simulink library "CompartmentsLib"  (Simulink 7.7)
settings: Solver=ode45  SolverMode=SingleTasking  StartTime=0.0  StopTime=10.0  RelTol=1e-3
undefined symbols (not defined in the file or in its folder): C, d, EK, EL, ENa, gA, gK, gL, gNa, L, magnitude, PSoma1, V0, VR
libraries: CurrentsLib x11, simulink x5, CompartmentsLib x2
settings Model: Creator=jpalma  LastModifiedBy=jpalma

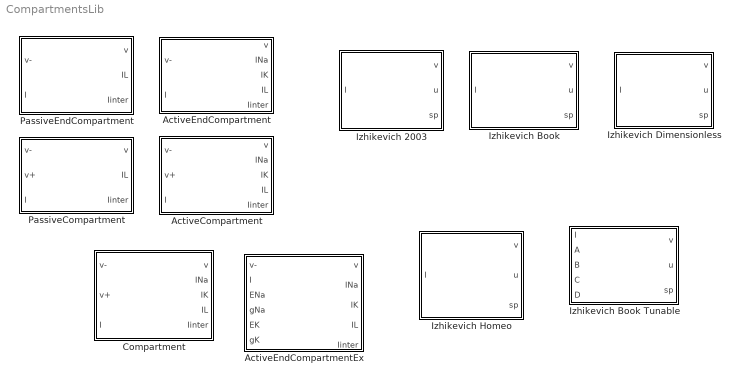
== system CompartmentsLib ==
  ActiveCompartment : Subsystem  mask{C=PSoma1(1), V0=PSoma1(2), gA=PSoma1(9), d=PSoma1(10), L=PSoma1(11), gNa=PSoma1(3), ENa=PSoma1(4), gK=PSoma1(5), EK=PSoma1(6), gL=PSoma1(7), EL=PSoma1(8)}
      mask prompts: C "Capacitance, C"; V0 "Initial Voltage, V0"; gA "Axial Conductance, gA"; d "Comp Diameter, d"; L "Comp Length, L"; gNa "Na Conductance, gNa"; ENa "Na Eq Voltage, ENa"; gK "K Conductance, gK"; EK "K Eq Voltage, EK"; gL "Leak Conductance, gL"; EL "Leak Eq Voltage, EL"
      mask help: Author: Jesse Palma
      mask Help: Author: Jesse Palma
      mask TabNameString: Basics,Basics,Basics,Basics,Basics,Currents,Currents,Currents,Currents,Currents,Currents
      mask Display: image(imread('../Libs/icons/Compartment.jpg'),'center');
  ActiveEndCompartment : Subsystem  mask{C=C, V0=V0, gA=gA, d=d, L=L, gNa=gNa, ENa=ENa, gK=gK, EK=EK, gL=gL, EL=EL}
      mask prompts: C "Capacitance, C"; V0 "Initial Voltage, V0"; gA "Axial Conductance, gA"; d "Comp Diameter, d"; L "Comp Length, L"; gNa "Na Conductance, gNa"; ENa "Na Eq Voltage, ENa"; gK "K Conductance, gK"; EK "K Eq Voltage, EK"; gL "Leak Conductance, gL"; EL "Leak Eq Voltage, EL"
      mask help: Author: Jesse Palma
      mask Help: Author: Jesse Palma
      mask TabNameString: Basic,Basic,Basic,Basic,Basic,Currents,Currents,Currents,Currents,Currents,Currents
      mask Display: image(imread('../Libs/icons/Compartment.jpg'),'center');
  ActiveEndCompartmentEx : Subsystem  mask{C=C, V0=V0, gA=gA, d=d, L=L, gL=gL, EL=EL}
      mask prompts: C "Capacitance, C"; V0 "Initial Voltage, V0"; gA "Axial Conductance, gA"; d "Comp Diameter, d"; L "Comp Length, L"; gL "Leak Conductance, gL"; EL "Leak Eq Voltage, EL"
      mask help: Author: Jesse Palma
      mask Help: Author: Jesse Palma
      mask TabNameString: Basic,Basic,Basic,Basic,Basic,Currents,Currents
      mask Display: image(imread('../Libs/icons/Compartment.jpg'),'center');
  Compartment : Subsystem  BlockChoice=ActiveEndCompartment  mask{ifEnd=on, ifActive=on, settings=UserDefined, C=1, V0=-65, gNa=45, ENa=50, gK=16, EK=-100, gL=0.03, EL=-60, gA=0.25, d=0.06, L=0.4}
      mask prompts: ifEnd "End Compartment"; ifActive "Active Compartment (Na and K)"; settings "Parameters Settings"; C "Capacitance"; V0 "Initial Voltage"; gNa "Na Conductance"; ENa "Na Eq Voltage"; gK "K Conductance"; EK "K Eq Voltage"; gL "Leak Conductance"; EL "Leak Eq Voltage"; gA "Axial Conductance"; d "Compartment Diameter"; L "Compartment Length"
      mask help: Author: Jesse Palma
      mask init:
      | maskStr = get_param(gcb,'MaskValues');
      | if (ifActive)
      |     if (ifEnd)
      |         BlockChoice = 'ActiveEndCompartment';
      |     else
      |         BlockChoice = 'ActiveCompartment';
      |     end
      | else
      |     if (ifEnd)
      |         BlockChoice = 'PassiveEndCompartment';
      |     else
      |         BlockChoice = 'PassiveCompartment';
      |     end
      | end
      | set_param([gcb], 'BlockChoice', BlockChoice);
      settings: TemplateBlock=self  MemberBlocks=ActiveCompartment,ActiveEndCompartment,PassiveCompartment,PassiveEndCompartment
      mask Help: Author: Jesse Palma
      mask StyleString: checkbox,checkbox,popup(Default1|UserDefined),edit,edit,edit,edit,edit,edit,edit,edit,edit,edit,edit
      mask CallbackString:
      | |maskStr = get_param(gcb,'MaskValues');
      | if strcmp(maskStr{2},'on')
      |     set_param(gcb,'MaskVisibilities',{'on';'on';'on';'on';'on';'on';'on';'on';'on';'on';'on';'on';'on';'on'});
      | else
      |     set_param(gcb,'MaskVisibilities',{'on';'on';'on';'on';'on';'off';'off';'off';'off';'on';'on';'on';'on';'on'});
      | end|maskStr = get_param(gcb,'MaskValues');
      | if strcmp(maskStr{3},'Default1')
      |    maskStr = get_param(gcb,'MaskValues');
      |    maskStr{4} = '1';
      |    maskStr{5} = '-65';
      |    maskStr{6} = '45';
      |    maskStr{7} = '50';
      |    maskStr{8} = '16';
      |    maskStr{9} = '-100';
      |    maskStr{10} = '0.03';
      |    maskStr{11} = '-60';
      |    maskStr{12} = '0.25';
      |    maskStr{13} = '0.06';
      |    maskStr{14} = '0.4';
      |    set_param(gcb, 'MaskValues', maskStr);
      | else
      | end|maskStr = get_param(gcb,'MaskValues');
      | maskStr{3} = 'UserDefined';
      | set_param(gcb, 'MaskValues', maskStr);|maskStr = get_param(gcb,'MaskValues');
      | maskStr{3} = 'UserDefined';
      | set_param(gcb, 'MaskValues', maskStr);|maskStr = get_param(gcb,'MaskValues');
      | maskStr{3} = 'UserDefined';
      | set_param(gcb, 'MaskValues', maskStr);|maskStr = get_param(gcb,'MaskValues');
      | maskStr{3} = 'UserDefined';
      | set_param(gcb, 'MaskValues', maskStr);|maskStr = get_param(gcb,'MaskValues');
      | maskStr{3} = 'UserDefined';
      | set_param(gcb, 'MaskValues', maskStr);|maskStr = get_param(gcb,'MaskValues');
      | maskStr{3} = 'UserDefined';
      | set_param(gcb, 'MaskValues', maskStr);|maskStr = get_param(gcb,'MaskValues');
      | maskStr{3} = 'UserDefined';
      | set_param(gcb, 'MaskValues', maskStr);|maskStr = get_param(gcb,'MaskValues');
      | maskStr{3} = 'UserDefined';
      | set_param(gcb, 'MaskValues', maskStr);|maskStr = get_param(gcb,'MaskValues');
      | maskStr{3} = 'UserDefined';
      | set_param(gcb, 'MaskValues', maskStr);|maskStr = get_param(gcb,'MaskValues');
      | maskStr{3} = 'UserDefined';
      | set_param(gcb, 'MaskValues', maskStr);|maskStr = get_param(gcb,'MaskValues');
      | maskStr{3} = 'UserDefined';
      | set_param(gcb, 'MaskValues', maskStr);
      mask TabNameString: Basics,Basics,Basics,Basics,Basics,Currents,Currents,Currents,Currents,Currents,Currents,Geometry,Geometry,Geometry
      mask Display: image(imread('../Libs/icons/Compartment.jpg'),'center');
  Izhikevich 2003 : Subsystem  mask{settings=UserDefined, A=0.02, B=0.2, C=-65, D=8, P2=0.04, P1=5, P0=140, VP=30, V0=-70, U0=-20}
      mask prompts: settings "Parameter Settings"; A "a, recovery u time constant"; B "b, dynamics parameter"; C "c,  reset value v"; D "d, reset shift u"; P2 "P2, 2nd order term"; P1 "P1, 1st order term"; P0 "P0, constant term"; VP "Vp, voltage peak"; V0 "V0, initial v value"; U0 "U0, intial u value"
      mask help:
      | Model from Eugene Izhikevich's 2003 Paper
      |     (Equations 1, 2 & 3)
      | Also in Eugene Izhikevich's 2004 Paper
      |
      | Simulink Model Design: Jesse Palma
      mask init:
      | maskStr = get_param(gcb,'MaskValues');
      mask Help:
      | Model from Eugene Izhikevich's 2003 Paper
      | <br>(Equations 1, 2 & 3)
      | <br>Also in Eugene Izhikevich's 2004 Paper
      | <br><br>
      | Simulink Model Design: Jesse Palma
      mask StyleString: popup(Tonic-Spiking-I04|Phasic-Spiking-I04|Tonic-Bursting-I04|UserDefined),edit,edit,edit,edit,edit,edit,edit,edit,edit,edit
      mask CallbackString:
      | maskStr = get_param(gcb,'MaskValues');
      | if strcmp(maskStr{1},'Tonic-Spiking-I04')
      |    maskStr = get_param(gcb,'MaskValues');
      |    maskStr{2} = '0.02'; %A
      |    maskStr{3} = '0.2';  %B
      |    maskStr{4} = '-65';  %C
      |    maskStr{5} = '6';    %D
      |    maskStr{6} = '0.04'; %P2
      |    maskStr{7} = '5';    %P1
      |    maskStr{8} = '140';  %P0
      |    maskStr{9} = '30';   %VP
      |    maskStr{10} = '-70'; %V0
      |    maskStr{11} = '-20';  %U0
      |    set_param(gcb, 'MaskValues', maskStr);
      | end
      | if strcmp(maskStr{1},'Phasic-Spiking-I04')
      |    maskStr = get_param(gcb,'MaskValues');
      |    maskStr{2} = '0.02'; %A
      |    maskStr{3} = '0.25';  %B
      |    maskStr{4} = '-65';  %C
      |    maskStr{5} = '6';    %D
      |    maskStr{6} = '0.04'; %P2
      |    maskStr{7} = '5';    %P1
      |    maskStr{8} = '140';  %P0
      |    maskStr{9} = '30';   %VP
      |    maskStr{10} = '-70'; %V0
      |    maskStr{11} = '-20';  %U0
      |    set_param(gcb, 'MaskValues', maskStr);
      | end
      | if strcmp(maskStr{1},'Tonic-Bursting-I04')
      |    maskStr = get_param(gcb,'MaskValues');
      |    maskStr{2} = '0.02'; %A
      |    maskStr{3} = '0.2';  %B
      |    maskStr{4} = '-50';  %C
      |    maskStr{5} = '2';    %D
      |    maskStr{6} = '0.04'; %P2
      |    maskStr{7} = '5';    %P1
      |    maskStr{8} = '140';  %P0
      |    maskStr{9} = '30';   %VP
      |    maskStr{10} = '-70'; %V0
      |    maskStr{11} = '-20';  %U0
      |    set_param(gcb, 'MaskValues', maskStr);
      | end|maskStr = get_param(gcb,'MaskValues');
      | maskStr{1} = 'UserDefined';
      | set_param(gcb, 'MaskValues', maskStr);|maskStr = get_param(gcb,'MaskValues');
      | maskStr{1} = 'UserDefined';
      | set_param(gcb, 'MaskValues', maskStr);|maskStr = get_param(gcb,'MaskValues');
      | maskStr{1} = 'UserDefined';
      | set_param(gcb, 'MaskValues', maskStr);|maskStr = get_param(gcb,'MaskValues');
      | maskStr{1} = 'UserDefined';
      | set_param(gcb, 'MaskValues', maskStr);|maskStr = get_param(gcb,'MaskValues');
      | maskStr{1} = 'UserDefined';
      | set_param(gcb, 'MaskValues', maskStr);|maskStr = get_param(gcb,'MaskValues');
      | maskStr{1} = 'UserDefined';
      | set_param(gcb, 'MaskValues', maskStr);|maskStr = get_param(gcb,'MaskValues');
      | maskStr{1} = 'UserDefined';
      | set_param(gcb, 'MaskValues', maskStr);|maskStr = get_param(gcb,'MaskValues');
      | maskStr{1} = 'UserDefined';
      | set_param(gcb, 'MaskValues', maskStr);|maskStr = get_param(gcb,'MaskValues');
      | maskStr{1} = 'UserDefined';
      | set_param(gcb, 'MaskValues', maskStr);|maskStr = get_param(gcb,'MaskValues');
      | maskStr{1} = 'UserDefined';
      | set_param(gcb, 'MaskValues', maskStr);
      mask Display: image(imread('../Libs/icons/Izhik.jpg'),'center');
  Izhikevich Book : Subsystem  mask{settings=UserDefined, A=0.03, B=-2, C=-50, D=100, CP=100, K=0.7, VR=-60, VT=-40, VP=35, V0=-60, U0=0}
      mask prompts: settings "Parameter Settings"; A "a, recovery u time constant"; B "b, dynamics parameter"; C "c,  reset value v"; D "d, reset shift u"; CP "Cp, capacitance"; VR "Vr, voltage rest"; VT "Vt, voltage threshold"; VP "Vpeak, voltage peak reset"; V0 "V0, initial v value"; U0 "U0, initial u value"
      mask help:
      | Model from Eugene Izhikevich's book "Dynamical Systems in Neuroscience"
      |     (Equations 8.5 & 8.6 on page 273)
      | 9 Paramters are reducable to 4-parameter model.
      |
      | Simulink Model Design: Jesse Palma
      mask Help:
      | Model from Eugene Izhikevich's book
      | <a href=http://www.izhikevich.org/publications/dsn/index.htm>"Dynamical Systems in Neuroscience"</a>
      | <br>(Equations 8.5 & 8.6 on page 273)<br>
      | 9 Paramters are reducable to 4-parameter model.
      | <br><br>
      | Simulink Model Design: Jesse Palma
      mask StyleString: popup(Regular-Spiking(p274-283)|Motor(p287)|UserDefined),edit,edit,edit,edit,edit,edit,edit,edit,edit,edit,edit
      mask CallbackString:
      | maskStr = get_param(gcb,'MaskValues');
      | if strcmp(maskStr{1},'Regular-Spiking(p274-283)')
      |    maskStr = get_param(gcb,'MaskValues');
      |    maskStr{2} = '0.03'; %A
      |    maskStr{3} = '-2';   %B
      |    maskStr{4} = '-50';  %C
      |    maskStr{5} = '100';  %D
      |    maskStr{6} = '100';  %CP
      |    maskStr{7} = '0.7';  %K
      |    maskStr{8} = '-60';  %VR
      |    maskStr{9} = '-40';  %VT
      |    maskStr{10} = '35';  %VP
      |    maskStr{11} = '-60'; %V0
      |    maskStr{12} = '0';   %U0
      |    set_param(gcb, 'MaskValues', maskStr);
      | end
      | if strcmp(maskStr{1},'Motor(p287)')
      |    maskStr = get_param(gcb,'MaskValues');
      |    maskStr{2} = '0.01'; %A
      |    maskStr{3} = '-0.25';%B
      |    maskStr{4} = '-40';  %C
      |    maskStr{5} = '90';   %D
      |    maskStr{6} = '30';   %CP
      |    maskStr{7} = '3';    %K
      |    maskStr{8} = '-55';  %VR
      |    maskStr{9} = '-42';  %VT
      |    maskStr{10} = '10';  %VP
      |    maskStr{11} = '-55'; %V0
      |    maskStr{12} = '0';   %U0
      |    set_param(gcb, 'MaskValues', maskStr);
      | end|maskStr = get_param(gcb,'MaskValues');
      | maskStr{1} = 'UserDefined';
      | set_param(gcb, 'MaskValues', maskStr);|maskStr = get_param(gcb,'MaskValues');
      | maskStr{1} = 'UserDefined';
      | set_param(gcb, 'MaskValues', maskStr);|maskStr = get_param(gcb,'MaskValues');
      | maskStr{1} = 'UserDefined';
      | set_param(gcb, 'MaskValues', maskStr);|maskStr = get_param(gcb,'MaskValues');
      | maskStr{1} = 'UserDefined';
      | set_param(gcb, 'MaskValues', maskStr);|maskStr = get_param(gcb,'MaskValues');
      | maskStr{1} = 'UserDefined';
      | set_param(gcb, 'MaskValues', maskStr);|maskStr = get_param(gcb,'MaskValues');
      | maskStr{1} = 'UserDefined';
      | set_param(gcb, 'MaskValues', maskStr);|maskStr = get_param(gcb,'MaskValues');
      | maskStr{1} = 'UserDefined';
      | set_param(gcb, 'MaskValues', maskStr);|maskStr = get_param(gcb,'MaskValues');
      | maskStr{1} = 'UserDefined';
      | set_param(gcb, 'MaskValues', maskStr);|maskStr = get_param(gcb,'MaskValues');
      | maskStr{1} = 'UserDefined';
      | set_param(gcb, 'MaskValues', maskStr);|maskStr = get_param(gcb,'MaskValues');
      | maskStr{1} = 'UserDefined';
      | set_param(gcb, 'MaskValues', maskStr);|maskStr = get_param(gcb,'MaskValues');
      | maskStr{1} = 'UserDefined';
      | set_param(gcb, 'MaskValues', maskStr);
      mask Display: image(imread('../Libs/icons/Izhik.jpg'),'center');
  "Izhikevich Book Tunable " : Subsystem  mask{settings=UserDefined, A=0.03, B=-2, C=-50, D=100, CP=100, K=0.7, VR=-60, VT=-40, VP=35, V0=-60, U0=0}
      mask prompts: settings "Parameter Settings"; A "a, recovery u time constant"; B "b, dynamics parameter"; C "c,  reset value v"; D "d, reset shift u"; CP "Cp, capacitance"; VR "Vr, voltage rest"; VT "Vt, voltage threshold"; VP "Vpeak, voltage peak reset"; V0 "V0, initial v value"; U0 "U0, initial u value"
      mask help:
      | Model from Eugene Izhikevich's book "Dynamical Systems in Neuroscience"
      |     (Equations 8.5 & 8.6 on page 273)
      | 9 Paramters are reducable to 4-parameter model.
      |
      | Simulink Model Design: Jesse Palma
      mask Help:
      | Model from Eugene Izhikevich's book
      | <a href=http://www.izhikevich.org/publications/dsn/index.htm>"Dynamical Systems in Neuroscience"</a>
      | <br>(Equations 8.5 & 8.6 on page 273)<br>
      | 9 Paramters are reducable to 4-parameter model.
      | <br><br>
      | Simulink Model Design: Jesse Palma
      mask StyleString: popup(Regular-Spiking(p274-283)|Motor(p287)|UserDefined),edit,edit,edit,edit,edit,edit,edit,edit,edit,edit,edit
      mask CallbackString:
      | maskStr = get_param(gcb,'MaskValues');
      | if strcmp(maskStr{1},'Regular-Spiking(p274-283)')
      |    maskStr = get_param(gcb,'MaskValues');
      |    maskStr{2} = '0.03'; %A
      |    maskStr{3} = '-2';   %B
      |    maskStr{4} = '-50';  %C
      |    maskStr{5} = '100';  %D
      |    maskStr{6} = '100';  %CP
      |    maskStr{7} = '0.7';  %K
      |    maskStr{8} = '-60';  %VR
      |    maskStr{9} = '-40';  %VT
      |    maskStr{10} = '35';  %VP
      |    maskStr{11} = '-60'; %V0
      |    maskStr{12} = '0';   %U0
      |    set_param(gcb, 'MaskValues', maskStr);
      | end
      | if strcmp(maskStr{1},'Motor(p287)')
      |    maskStr = get_param(gcb,'MaskValues');
      |    maskStr{2} = '0.01'; %A
      |    maskStr{3} = '-0.25';%B
      |    maskStr{4} = '-40';  %C
      |    maskStr{5} = '90';   %D
      |    maskStr{6} = '30';   %CP
      |    maskStr{7} = '3';    %K
      |    maskStr{8} = '-55';  %VR
      |    maskStr{9} = '-42';  %VT
      |    maskStr{10} = '10';  %VP
      |    maskStr{11} = '-55'; %V0
      |    maskStr{12} = '0';   %U0
      |    set_param(gcb, 'MaskValues', maskStr);
      | end|maskStr = get_param(gcb,'MaskValues');
      | maskStr{1} = 'UserDefined';
      | set_param(gcb, 'MaskValues', maskStr);|maskStr = get_param(gcb,'MaskValues');
      | maskStr{1} = 'UserDefined';
      | set_param(gcb, 'MaskValues', maskStr);|maskStr = get_param(gcb,'MaskValues');
      | maskStr{1} = 'UserDefined';
      | set_param(gcb, 'MaskValues', maskStr);|maskStr = get_param(gcb,'MaskValues');
      | maskStr{1} = 'UserDefined';
      | set_param(gcb, 'MaskValues', maskStr);|maskStr = get_param(gcb,'MaskValues');
      | maskStr{1} = 'UserDefined';
      | set_param(gcb, 'MaskValues', maskStr);|maskStr = get_param(gcb,'MaskValues');
      | maskStr{1} = 'UserDefined';
      | set_param(gcb, 'MaskValues', maskStr);|maskStr = get_param(gcb,'MaskValues');
      | maskStr{1} = 'UserDefined';
      | set_param(gcb, 'MaskValues', maskStr);|maskStr = get_param(gcb,'MaskValues');
      | maskStr{1} = 'UserDefined';
      | set_param(gcb, 'MaskValues', maskStr);|maskStr = get_param(gcb,'MaskValues');
      | maskStr{1} = 'UserDefined';
      | set_param(gcb, 'MaskValues', maskStr);|maskStr = get_param(gcb,'MaskValues');
      | maskStr{1} = 'UserDefined';
      | set_param(gcb, 'MaskValues', maskStr);|maskStr = get_param(gcb,'MaskValues');
      | maskStr{1} = 'UserDefined';
      | set_param(gcb, 'MaskValues', maskStr);
      mask Display: image(imread('../Libs/icons/Izhik.jpg'),'center');
  Izhikevich Dimensionless : Subsystem  mask{settings=UserDefined, A=1, B=1, C=1, D=1, V0=0, U0=0}
      mask prompts: settings "Parameter Settings"; A "a, recovery u time constant"; B "b, dynamics parameter"; C "c,  reset value v"; D "d, reset shift u"; V0 "V0, initial v value"; U0 "U0, initial u value"
      mask help:
      | Dimensionless Model from Eugene Izhikevich's book "Dynamical Systems in Neuroscience"
      |     (Equations 8.3 & 8.4 on page 273)
      |
      | Simulink Model Design: Jesse Palma
      mask init:
      | maskStr = get_param(gcb,'MaskValues');
      mask Help:
      | Dimensionless Model from Eugene Izhikevich's book "Dynamical Systems in Neuroscience"
      |     (Equations 8.3 & 8.4 on page 273)
      | 
      | Simulink Model Design: Jesse Palma
      mask StyleString: popup(Default1|UserDefined),edit,edit,edit,edit,edit,edit
      mask CallbackString:
      | maskStr = get_param(gcb,'MaskValues');
      | if strcmp(maskStr{1},'Default1')
      |    maskStr = get_param(gcb,'MaskValues');
      |    maskStr{2} = '1';
      |    maskStr{3} = '1';
      |    maskStr{4} = '1';
      |    maskStr{5} = '1';
      |    maskStr{6} = '0';
      |    maskStr{7} = '0';
      |    set_param(gcb, 'MaskValues', maskStr);
      | else
      | end|maskStr = get_param(gcb,'MaskValues');
      | maskStr{1} = 'UserDefined';
      | set_param(gcb, 'MaskValues', maskStr);|maskStr = get_param(gcb,'MaskValues');
      | maskStr{1} = 'UserDefined';
      | set_param(gcb, 'MaskValues', maskStr);|maskStr = get_param(gcb,'MaskValues');
      | maskStr{1} = 'UserDefined';
      | set_param(gcb, 'MaskValues', maskStr);|maskStr = get_param(gcb,'MaskValues');
      | maskStr{1} = 'UserDefined';
      | set_param(gcb, 'MaskValues', maskStr);|maskStr = get_param(gcb,'MaskValues');
      | maskStr{1} = 'UserDefined';
      | set_param(gcb, 'MaskValues', maskStr);|maskStr = get_param(gcb,'MaskValues');
      | maskStr{1} = 'UserDefined';
      | set_param(gcb, 'MaskValues', maskStr);
      mask Display: image(imread('../Libs/icons/Izhik.jpg'),'center');
  Izhikevich Homeo : Subsystem
      mask Display: image(imread('../Libs/icons/Izhik.jpg'),'center');
  PassiveCompartment : Subsystem  mask{C=C, V0=V0, gA=gA, d=d, L=L, gL=gL, EL=EL}
      mask prompts: C "Capacitance, C"; V0 "Initial Voltage, V0"; gA "Axial Conductance, gA"; d "Comp Diameter, d"; L "Comp Length, L"; gL "Leak Conductance, gL"; EL "Leak Eq Voltage, EL"
      mask help: Author: Jesse Palma
      mask Help: Author: Jesse Palma
      mask TabNameString: Basics,Basics,Basics,Basics,Basics,Currents,Currents
      mask Display: image(imread('../Libs/icons/Compartment.jpg'),'center');
  PassiveEndCompartment : Subsystem  mask{C=C, V0=V0, gA=gA, d=d, L=L, gL=gL, EL=EL}
      mask prompts: C "Capacitance, C"; V0 "Initial Voltage, V0"; gA "Axial Conductance, gA"; d "Comp Diameter, d"; L "Comp Length, L"; gL "Leak Conductance, gL"; EL "Leak Eq Voltage, EL"
      mask help: Author: Jesse Palma
      mask Help: Author: Jesse Palma
      mask TabNameString: Basic,Basic,Basic,Basic,Basic,Currents,Currents
      mask Display: image(imread('../Libs/icons/Compartment.jpg'),'center');

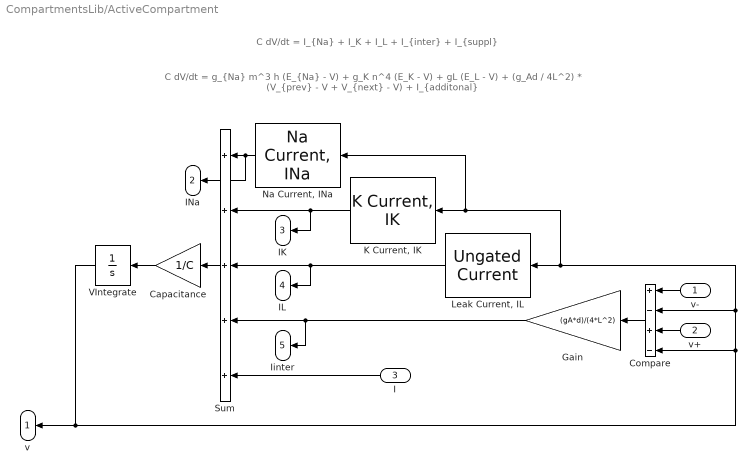
== system CompartmentsLib/ActiveCompartment ==
  note: C dV/dt = I_{Na} + I_K + I_L + I_{inter} + I_{suppl}
  note: C dV/dt = g_{Na} m^3 h (E_{Na} - V) + g_K n^4 (E_K - V) + gL (E_L - V) + (g_Ad / 4L^2) * (V_{prev} - V + V_{next} - V) + I_{additonal}
  v- : Inport
  v+ : Inport  Port=2
  I : Inport  Port=3
  Capacitance : Gain  Gain=1/C
  Compare : Sum  Inputs=+-+-
  Gain : Gain  Gain=(gA*d)/(4*L^2)
  "K Current, IK" : CurrentsLib/K Current, IK  SystemSampleTime=-1  EK=EK  gK=gK  n_a=n3_alpha  n_b=n3_beta
  "Leak Current, IL" : CurrentsLib/Ungated Current  SystemSampleTime=-1  EX=EL  gX=gL
  "Na Current, INa" : CurrentsLib/Na Current, INa  SystemSampleTime=-1  ENa=ENa  gNa=gNa  m_a=m3_alpha  m_b=m3_beta  h_a=h3_alpha  h_b=h3_beta
  Sum : Sum  Inputs=+++++
  VIntegrate : Integrator  InitialCondition=V0
  v : Outport
  INa : Outport  Port=2
  IK : Outport  Port=3
  IL : Outport  Port=4
  Iinter : Outport  Port=5
  wires:
  "K Current, IK"/1 -> IK/1, Sum/2
  "Na Current, INa"/1 -> INa/1, Sum/1
  Gain/1 -> Sum/4, Iinter/1
  I/1 -> Sum/5
  VIntegrate/1 -> v/1, "Na Current, INa"/1, "K Current, IK"/1, "Leak Current, IL"/1, Compare/2, Compare/4
  Capacitance/1 -> VIntegrate/1
  Sum/1 -> Capacitance/1
  "Leak Current, IL"/1 -> IL/1, Sum/3
  Compare/1 -> Gain/1
  v-/1 -> Compare/1
  v+/1 -> Compare/3

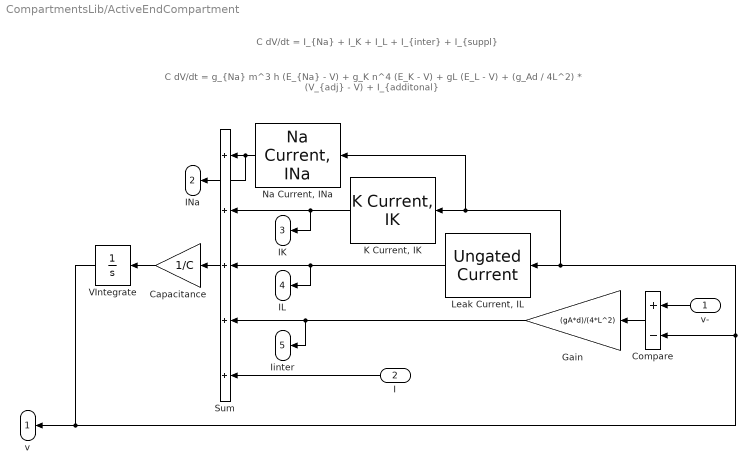
== system CompartmentsLib/ActiveEndCompartment ==
  note: C dV/dt = g_{Na} m^3 h (E_{Na} - V) + g_K n^4 (E_K - V) + gL (E_L - V) + (g_Ad / 4L^2) * (V_{adj} - V) + I_{additonal}
  note: C dV/dt = I_{Na} + I_K + I_L + I_{inter} + I_{suppl}
  v- : Inport
  I : Inport  Port=2
  Capacitance : Gain  Gain=1/C
  Compare : Sum  Inputs=+-
  Gain : Gain  Gain=(gA*d)/(4*L^2)
  "K Current, IK" : CurrentsLib/K Current, IK  SystemSampleTime=-1  EK=EK  gK=gK  n_a=n3_alpha  n_b=n3_beta
  "Leak Current, IL" : CurrentsLib/Ungated Current  SystemSampleTime=-1  EX=EL  gX=gL
  "Na Current, INa" : CurrentsLib/Na Current, INa  SystemSampleTime=-1  ENa=ENa  gNa=gNa  m_a=m3_alpha  m_b=m3_beta  h_a=h3_alpha  h_b=h3_beta
  Sum : Sum  Inputs=+++++
  VIntegrate : Integrator  InitialCondition=V0
  v : Outport
  INa : Outport  Port=2
  IK : Outport  Port=3
  IL : Outport  Port=4
  Iinter : Outport  Port=5
  wires:
  v-/1 -> Compare/1
  Compare/1 -> Gain/1
  "Leak Current, IL"/1 -> Sum/3, IL/1
  Sum/1 -> Capacitance/1
  Capacitance/1 -> VIntegrate/1
  VIntegrate/1 -> v/1, Compare/2, "Leak Current, IL"/1, "K Current, IK"/1, "Na Current, INa"/1
  I/1 -> Sum/5
  Gain/1 -> Iinter/1, Sum/4
  "Na Current, INa"/1 -> Sum/1, INa/1
  "K Current, IK"/1 -> Sum/2, IK/1

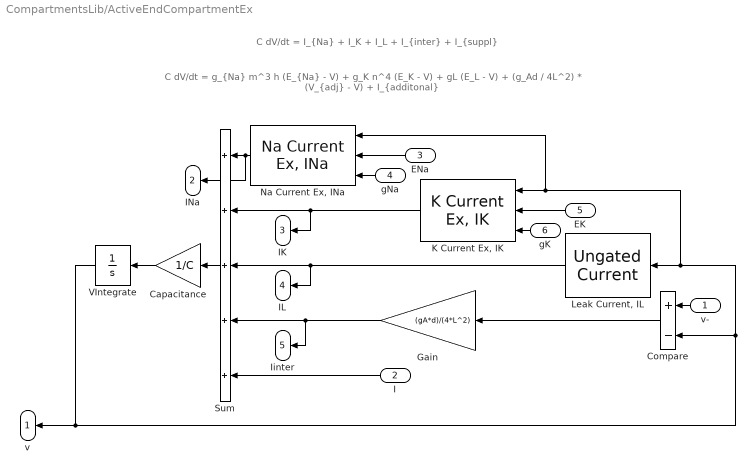
== system CompartmentsLib/ActiveEndCompartmentEx ==
  note: C dV/dt = I_{Na} + I_K + I_L + I_{inter} + I_{suppl}
  note: C dV/dt = g_{Na} m^3 h (E_{Na} - V) + g_K n^4 (E_K - V) + gL (E_L - V) + (g_Ad / 4L^2) * (V_{adj} - V) + I_{additonal}
  v- : Inport
  I : Inport  Port=2
  ENa : Inport  Port=3
  gNa : Inport  Port=4
  EK : Inport  Port=5
  gK : Inport  Port=6
  Capacitance : Gain  Gain=1/C
  Compare : Sum  Inputs=+-
  Gain : Gain  Gain=(gA*d)/(4*L^2)
  "K Current Ex, IK" : CurrentsLib/K Current Ex, IK  SystemSampleTime=-1  n_a=n3_alpha  n_b=n3_beta
  "Leak Current, IL" : CurrentsLib/Ungated Current  SystemSampleTime=-1  EX=EL  gX=gL
  "Na Current Ex, INa" : CurrentsLib/Na Current Ex, INa  SystemSampleTime=-1  m_a=m3_alpha  m_b=m3_beta  h_a=h3_alpha  h_b=h3_beta
  Sum : Sum  Inputs=+++++
  VIntegrate : Integrator  InitialCondition=V0
  v : Outport
  INa : Outport  Port=2
  IK : Outport  Port=3
  IL : Outport  Port=4
  Iinter : Outport  Port=5
  wires:
  "K Current Ex, IK"/1 -> IK/1, Sum/2
  "Na Current Ex, INa"/1 -> INa/1, Sum/1
  Gain/1 -> Sum/4, Iinter/1
  I/1 -> Sum/5
  VIntegrate/1 -> Compare/2, "Leak Current, IL"/1, "K Current Ex, IK"/1, "Na Current Ex, INa"/1, v/1
  Capacitance/1 -> VIntegrate/1
  Sum/1 -> Capacitance/1
  "Leak Current, IL"/1 -> IL/1, Sum/3
  Compare/1 -> Gain/1
  v-/1 -> Compare/1
  ENa/1 -> "Na Current Ex, INa"/2
  gNa/1 -> "Na Current Ex, INa"/3
  gK/1 -> "K Current Ex, IK"/3
  EK/1 -> "K Current Ex, IK"/2

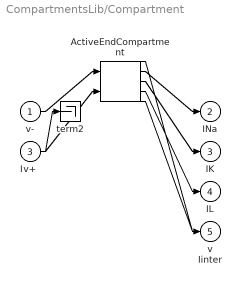
== system CompartmentsLib/Compartment ==
  v- : Inport
  v+ : Inport  Port=2
  I : Inport  Port=3
  ActiveEndCompartment : CompartmentsLib/ActiveEndCompartment  SystemSampleTime=-1  C=PSoma1(1)  V0=PSoma1(2)  gA=PSoma1(9)  d=PSoma1(10)  L=PSoma1(11)  gNa=PSoma1(3)  ENa=PSoma1(4)  gK=PSoma1(5)  EK=PSoma1(6)  gL=PSoma1(7)  EL=PSoma1(8)
  term2 : Terminator
  v : Outport
  INa : Outport  Port=2
  IK : Outport  Port=3
  IL : Outport  Port=4
  Iinter : Outport  Port=5
  wires:
  v-/1 -> ActiveEndCompartment/1
  I/1 -> ActiveEndCompartment/2
  ActiveEndCompartment/1 -> v/1
  ActiveEndCompartment/2 -> INa/1
  ActiveEndCompartment/3 -> IK/1
  ActiveEndCompartment/4 -> IL/1
  ActiveEndCompartment/5 -> Iinter/1
  v+/1 -> term2/1

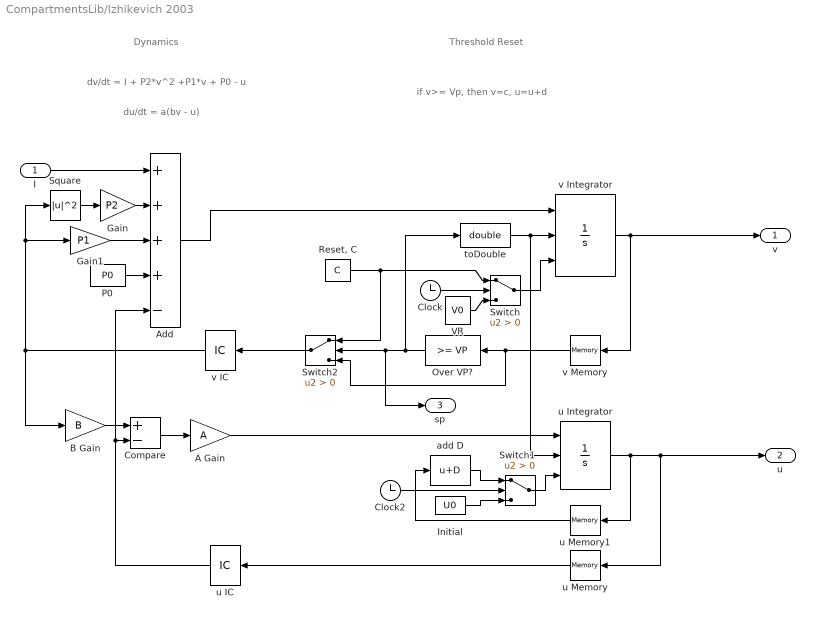
== system CompartmentsLib/Izhikevich 2003 ==
  note: dv/dt = I + P2*v^2 +P1*v + P0 - u
  note: du/dt = a(bv - u)
  note: if v>= Vp, then
      | v=c, u=u+d
  note: Dynamics
  note: Threshold Reset
  I : Inport
  " Initial" : Constant  Value=U0
  A Gain : Gain  Gain=A
  Add : Sum  Inputs=++++-
  B Gain : Gain  Gain=B
  Clock : Clock
      settings: Decimation=10
  Clock2 : Clock
      settings: Decimation=10
  Compare : Sum  Inputs=+-
  Gain : Gain  Gain=P2
  Gain1 : Gain  Gain=P1
  Over VP? : simulink/Logic and Bit Operations/Compare To Constant  SystemSampleTime=-1  relop=>=  const=VP  LogicOutDataTypeMode=boolean  ZeroCross=off
  P0 : Constant  Value=P0
  "Reset, C" : Constant  Value=C
  Square : Math  Operator=magnitude^2  SaturateOnIntegerOverflow=on
  Switch : Switch  Criteria=u2 > Threshold
  Switch1 : Switch  Criteria=u2 > Threshold
  Switch2 : Switch  Criteria=u2 > Threshold
  VR : Constant  Value=V0
  add D : Bias  Bias=D  SaturateOnIntegerOverflow=on
  toDouble : DataTypeConversion  OutDataTypeStr=double
  u IC : InitialCondition  Value=U0
  u Integrator : Integrator  ExternalReset=falling  InitialConditionSource=external
  u Memory : Memory
  u Memory1 : Memory
  v IC : InitialCondition  Value=V0
  v Integrator : Integrator  ExternalReset=rising  InitialConditionSource=external  InitialCondition=VR
  v Memory : Memory
  v : Outport
  u : Outport  Port=2
  sp : Outport  Port=3
  wires:
  u Memory1/1 -> add D/1
  add D/1 -> Switch1/1
  P0/1 -> Add/4
  VR/1 -> Switch/3
  Gain1/1 -> Add/3
  Gain/1 -> Add/2
  Square/1 -> Gain/1
  I/1 -> Add/1
  Add/1 -> v Integrator/1
  A Gain/1 -> u Integrator/1
  B Gain/1 -> Compare/1
  Compare/1 -> A Gain/1
  Over VP?/1 -> toDouble/1, Switch2/2, sp/1
  v Memory/1 -> Over VP?/1, Switch2/3
  " Initial"/1 -> Switch1/3
  Switch1/1 -> u Integrator/3
  Clock2/1 -> Switch1/2
  u Integrator/1 -> u Memory1/1, u Memory/1, u/1
  "Reset, C"/1 -> Switch2/1, Switch/1
  Clock/1 -> Switch/2
  Switch/1 -> v Integrator/3
  v Integrator/1 -> v/1, v Memory/1
  toDouble/1 -> u Integrator/2, v Integrator/2
  Switch2/1 -> v IC/1
  u Memory/1 -> u IC/1
  v IC/1 -> Gain1/1, Square/1, B Gain/1
  u IC/1 -> Add/5, Compare/2

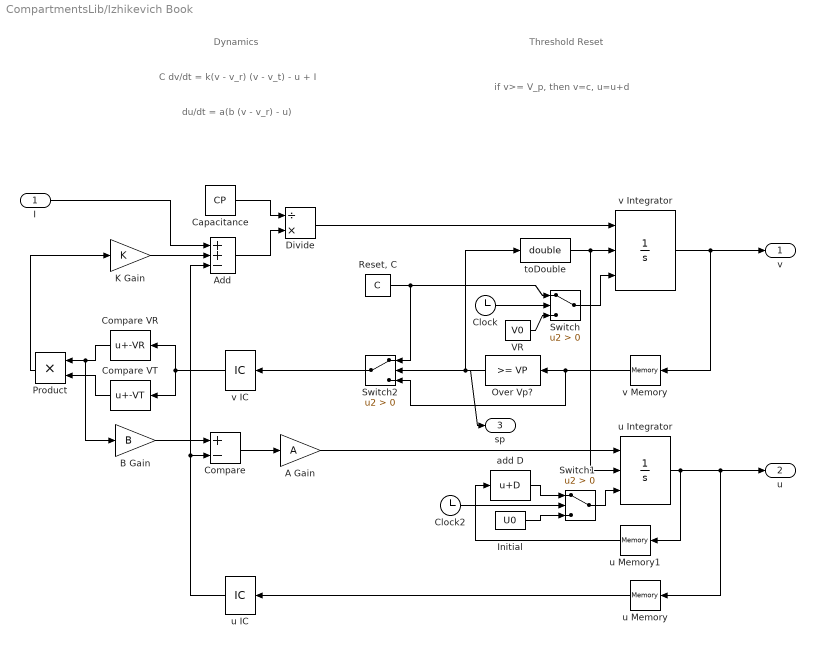
== system CompartmentsLib/Izhikevich Book ==
  note: Threshold Reset
  note: Dynamics
  note: if v>= V_p, then
      | v=c, u=u+d
  note: du/dt = a(b (v - v_r) - u)
  note: C dv/dt = k(v - v_r) (v - v_t) - u + I
  I : Inport
  " Initial" : Constant  Value=U0
  A Gain : Gain  Gain=A
  Add : Sum  Inputs=++-
  B Gain : Gain  Gain=B
  Capacitance : Constant  Value=CP
  Clock : Clock
      settings: Decimation=10
  Clock2 : Clock
      settings: Decimation=10
  Compare : Sum  Inputs=+-
  Compare VR : Bias  Bias=-VR
  Compare VT : Bias  Bias=-VT
  Divide : Product  Inputs=/*
  K Gain : Gain  Gain=K
  Over Vp? : simulink/Logic and Bit Operations/Compare To Constant  SystemSampleTime=-1  relop=>=  const=VP  LogicOutDataTypeMode=boolean  ZeroCross=off
  Product : Product  RndMeth=Zero
  "Reset, C" : Constant  Value=C
  Switch : Switch  Criteria=u2 > Threshold  ZeroCross=off
  Switch1 : Switch  Criteria=u2 > Threshold  ZeroCross=off
  Switch2 : Switch  Criteria=u2 > Threshold  ZeroCross=off
  VR : Constant  Value=V0
  add D : Bias  Bias=D
  toDouble : DataTypeConversion  OutDataTypeStr=double
  u IC : InitialCondition  Value=U0
  u Integrator : Integrator  ExternalReset=rising  InitialConditionSource=external  ZeroCross=off
  u Memory : Memory
  u Memory1 : Memory
  v IC : InitialCondition  Value=V0
  v Integrator : Integrator  ExternalReset=rising  InitialConditionSource=external  InitialCondition=VR  ZeroCross=off
  v Memory : Memory
  v : Outport
  u : Outport  Port=2
  sp : Outport  Port=3
  wires:
  Over Vp?/1 -> toDouble/1, Switch2/2, sp/1
  v Memory/1 -> Over Vp?/1, Switch2/3
  Switch2/1 -> v IC/1
  " Initial"/1 -> Switch1/3
  add D/1 -> Switch1/1
  Switch1/1 -> u Integrator/3
  Clock2/1 -> Switch1/2
  A Gain/1 -> u Integrator/1
  Divide/1 -> v Integrator/1
  u Integrator/1 -> u Memory/1, u/1, u Memory1/1
  "Reset, C"/1 -> Switch/1, Switch2/1
  Clock/1 -> Switch/2
  Switch/1 -> v Integrator/3
  u IC/1 -> Compare/2, Add/3
  v IC/1 -> Compare VR/1, Compare VT/1
  Compare/1 -> A Gain/1
  B Gain/1 -> Compare/1
  u Memory/1 -> u IC/1
  Product/1 -> K Gain/1
  I/1 -> Add/1
  Compare VR/1 -> Product/1, B Gain/1
  Compare VT/1 -> Product/2
  K Gain/1 -> Add/2
  v Integrator/1 -> v Memory/1, v/1
  toDouble/1 -> u Integrator/2, v Integrator/2
  Add/1 -> Divide/2
  Capacitance/1 -> Divide/1
  VR/1 -> Switch/3
  u Memory1/1 -> add D/1

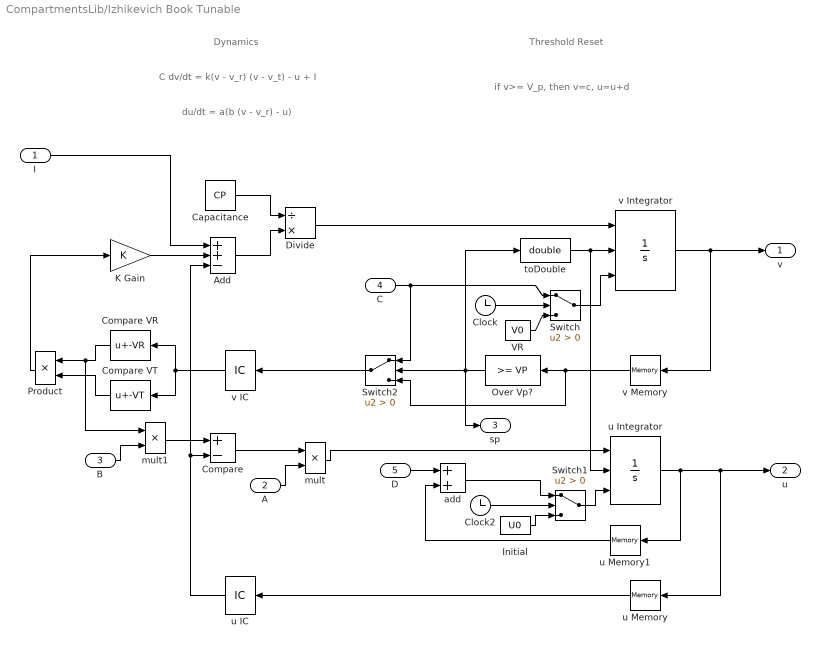
== system CompartmentsLib/Izhikevich Book Tunable  ==
  note: Threshold Reset
  note: Dynamics
  note: if v>= V_p, then
      | v=c, u=u+d
  note: du/dt = a(b (v - v_r) - u)
  note: C dv/dt = k(v - v_r) (v - v_t) - u + I
  I : Inport
  A : Inport  Port=2
  B : Inport  Port=3
  C : Inport  Port=4
  D : Inport  Port=5
  " Initial" : Constant  Value=U0
  Add : Sum  Inputs=++-
  Capacitance : Constant  Value=CP
  Clock : Clock
      settings: Decimation=10
  Clock2 : Clock
      settings: Decimation=10
  Compare : Sum  Inputs=+-
  Compare VR : Bias  Bias=-VR
  Compare VT : Bias  Bias=-VT
  Divide : Product  Inputs=/*
  K Gain : Gain  Gain=K
  Over Vp? : simulink/Logic and Bit Operations/Compare To Constant  SystemSampleTime=-1  relop=>=  const=VP  LogicOutDataTypeMode=boolean
  Product : Product  RndMeth=Zero
  Switch : Switch  Criteria=u2 > Threshold
  Switch1 : Switch  Criteria=u2 > Threshold
  Switch2 : Switch  Criteria=u2 > Threshold
  VR : Constant  Value=V0
  add : Sum
  mult : Product  Inputs=**
  mult1 : Product  Inputs=**
  toDouble : DataTypeConversion  OutDataTypeStr=double
  u IC : InitialCondition  Value=U0
  u Integrator : Integrator  ExternalReset=rising  InitialConditionSource=external  ZeroCross=off
  u Memory : Memory
  u Memory1 : Memory
  v IC : InitialCondition  Value=V0
  v Integrator : Integrator  ExternalReset=rising  InitialConditionSource=external  InitialCondition=VR  ZeroCross=off
  v Memory : Memory
  v : Outport
  u : Outport  Port=2
  sp : Outport  Port=3
  wires:
  Over Vp?/1 -> toDouble/1, Switch2/2, sp/1
  v Memory/1 -> Over Vp?/1, Switch2/3
  Switch2/1 -> v IC/1
  " Initial"/1 -> Switch1/3
  add/1 -> Switch1/1
  Switch1/1 -> u Integrator/3
  Clock2/1 -> Switch1/2
  mult/1 -> u Integrator/1
  Divide/1 -> v Integrator/1
  u Integrator/1 -> u Memory/1, u/1, u Memory1/1
  C/1 -> Switch/1, Switch2/1
  Clock/1 -> Switch/2
  Switch/1 -> v Integrator/3
  u IC/1 -> Compare/2, Add/3
  v IC/1 -> Compare VR/1, Compare VT/1
  mult1/1 -> Compare/1
  u Memory/1 -> u IC/1
  Product/1 -> K Gain/1
  I/1 -> Add/1
  Compare VR/1 -> Product/1, mult1/1
  Compare VT/1 -> Product/2
  K Gain/1 -> Add/2
  v Integrator/1 -> v Memory/1, v/1
  toDouble/1 -> u Integrator/2, v Integrator/2
  Add/1 -> Divide/2
  Capacitance/1 -> Divide/1
  VR/1 -> Switch/3
  u Memory1/1 -> add/2
  A/1 -> mult/2
  Compare/1 -> mult/1
  B/1 -> mult1/2
  D/1 -> add/1

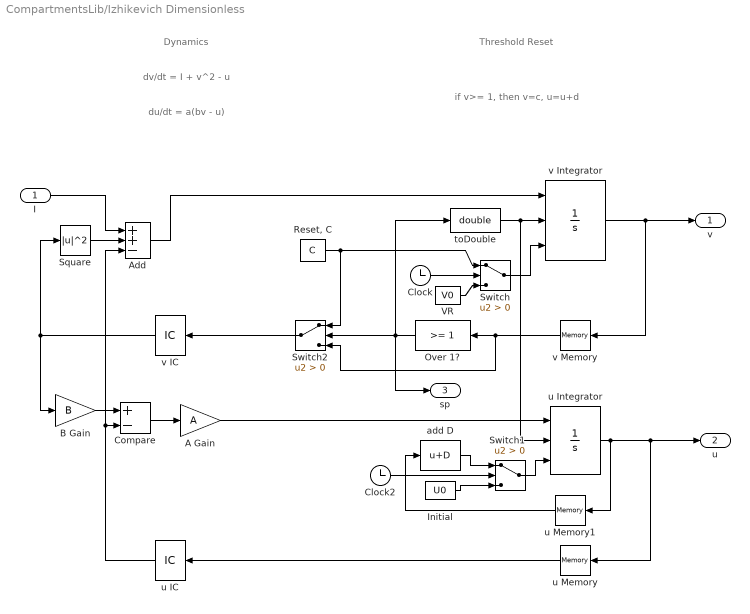
== system CompartmentsLib/Izhikevich Dimensionless ==
  note: dv/dt = I + v^2 - u
  note: du/dt = a(bv - u)
  note: if v>= 1, then
      | v=c, u=u+d
  note: Dynamics
  note: Threshold Reset
  I : Inport
  " Initial" : Constant  Value=U0
  A Gain : Gain  Gain=A
  Add : Sum  Inputs=++-
  B Gain : Gain  Gain=B
  Clock : Clock
      settings: Decimation=10
  Clock2 : Clock
      settings: Decimation=10
  Compare : Sum  Inputs=+-
  Over 1? : simulink/Logic and Bit Operations/Compare To Constant  SystemSampleTime=-1  relop=>=  const=1  LogicOutDataTypeMode=boolean  ZeroCross=off
  "Reset, C" : Constant  Value=C
  Square : Math  Operator=magnitude^2  SaturateOnIntegerOverflow=on
  Switch : Switch  Criteria=u2 > Threshold
  Switch1 : Switch  Criteria=u2 > Threshold
  Switch2 : Switch  Criteria=u2 > Threshold
  VR : Constant  Value=V0
  add D : Bias  Bias=D
  toDouble : DataTypeConversion  OutDataTypeStr=double
  u IC : InitialCondition  Value=U0
  u Integrator : Integrator  ExternalReset=rising  InitialConditionSource=external
  u Memory : Memory
  u Memory1 : Memory
  v IC : InitialCondition  Value=V0
  v Integrator : Integrator  ExternalReset=rising  InitialConditionSource=external  InitialCondition=VR
  v Memory : Memory
  v : Outport
  u : Outport  Port=2
  sp : Outport  Port=3
  wires:
  I/1 -> Add/1
  Add/1 -> v Integrator/1
  Square/1 -> Add/2
  A Gain/1 -> u Integrator/1
  B Gain/1 -> Compare/1
  Compare/1 -> A Gain/1
  Over 1?/1 -> Switch2/2, toDouble/1, sp/1
  v Memory/1 -> Over 1?/1, Switch2/3
  " Initial"/1 -> Switch1/3
  add D/1 -> Switch1/1
  Switch1/1 -> u Integrator/3
  Clock2/1 -> Switch1/2
  u Integrator/1 -> u Memory/1, u/1, u Memory1/1
  "Reset, C"/1 -> Switch/1, Switch2/1
  Clock/1 -> Switch/2
  Switch/1 -> v Integrator/3
  v Integrator/1 -> v Memory/1, v/1
  toDouble/1 -> u Integrator/2, v Integrator/2
  Switch2/1 -> v IC/1
  u Memory/1 -> u IC/1
  v IC/1 -> Square/1, B Gain/1
  u IC/1 -> Add/3, Compare/2
  VR/1 -> Switch/3
  u Memory1/1 -> add D/1

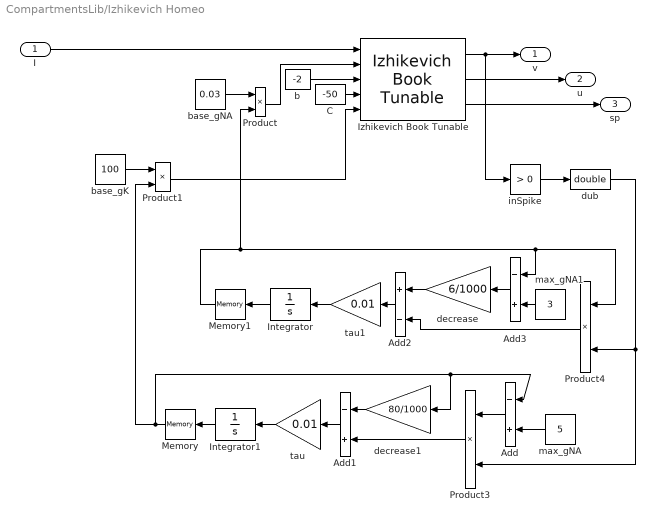
== system CompartmentsLib/Izhikevich Homeo ==
  I : Inport
  Add : Sum  Inputs=-+
  Add1 : Sum  Inputs=-+
  Add2 : Sum  Inputs=+-
  Add3 : Sum  Inputs=-+
  C : Constant  Value=-50
  Integrator : Integrator  InitialCondition=1  LimitOutput=on  LowerSaturationLimit=0.001  ZeroCross=off
  Integrator1 : Integrator  InitialCondition=1  LimitOutput=on  LowerSaturationLimit=0.001  ZeroCross=off
  "Izhikevich Book Tunable " : CompartmentsLib/Izhikevich Book Tunable   SystemSampleTime=-1  settings=UserDefined  A=0.03  B=-2  C=-50  D=100  CP=100  K=0.7  VR=-60  VT=-40  VP=35  V0=-60  U0=0
  Memory : Memory
  Memory1 : Memory
  Product{,1,3..4} (4 alike) : Product  RndMeth=Zero
  b : Constant  Value=-2
  base_gK : Constant  Value=100
  base_gNA : Constant  Value=0.03
  decrease : Gain  Gain=6/1000
  decrease1 : Gain  Gain=80/1000
  dub : DataTypeConversion  OutDataTypeStr=double
  inSpike : simulink/Logic and Bit Operations/Compare To Constant  SystemSampleTime=-1  relop=>  const=0  LogicOutDataTypeMode=uint8
  max_gNA : Constant  Value=5
  max_gNA1 : Constant  Value=3
  tau : Gain  Gain=0.01
  tau1 : Gain  Gain=0.01
  v : Outport
  u : Outport  Port=2
  sp : Outport  Port=3
  wires:
  C/1 -> "Izhikevich Book Tunable "/4
  base_gNA/1 -> Product/1
  base_gK/1 -> Product1/1
  inSpike/1 -> dub/1
  Add2/1 -> tau1/1
  tau1/1 -> Integrator/1
  dub/1 -> Product3/2, Product4/2
  Integrator/1 -> Memory1/1
  Integrator1/1 -> Memory/1
  Memory/1 -> decrease1/1, Add/1, Product1/2
  Add1/1 -> tau/1
  Product3/1 -> Add1/2
  max_gNA/1 -> Add/2
  tau/1 -> Integrator1/1
  Memory1/1 -> Add3/1, Product4/1, Product/2
  Product4/1 -> Add2/2
  max_gNA1/1 -> Add3/2
  decrease/1 -> Add2/1
  decrease1/1 -> Add1/1
  Add3/1 -> decrease/1
  Add/1 -> Product3/1
  Product/1 -> "Izhikevich Book Tunable "/2
  Product1/1 -> "Izhikevich Book Tunable "/5
  b/1 -> "Izhikevich Book Tunable "/3
  "Izhikevich Book Tunable "/1 -> inSpike/1, v/1
  I/1 -> "Izhikevich Book Tunable "/1
  "Izhikevich Book Tunable "/2 -> u/1
  "Izhikevich Book Tunable "/3 -> sp/1

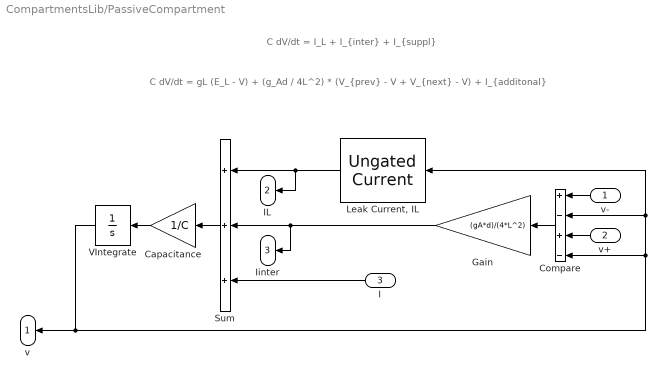
== system CompartmentsLib/PassiveCompartment ==
  note: C dV/dt = gL (E_L - V) + (g_Ad / 4L^2) * (V_{prev} - V + V_{next} - V) + I_{additonal}
  note: C dV/dt = I_L + I_{inter} + I_{suppl}
  v- : Inport
  v+ : Inport  Port=2
  I : Inport  Port=3
  Capacitance : Gain  Gain=1/C
  Compare : Sum  Inputs=+-+-
  Gain : Gain  Gain=(gA*d)/(4*L^2)
  "Leak Current, IL" : CurrentsLib/Ungated Current  SystemSampleTime=-1  EX=EL  gX=gL
  Sum : Sum  Inputs=+++
  VIntegrate : Integrator  InitialCondition=V0
  v : Outport
  IL : Outport  Port=2
  Iinter : Outport  Port=3
  wires:
  v+/1 -> Compare/3
  v-/1 -> Compare/1
  Compare/1 -> Gain/1
  "Leak Current, IL"/1 -> IL/1, Sum/1
  Sum/1 -> Capacitance/1
  Capacitance/1 -> VIntegrate/1
  VIntegrate/1 -> Compare/4, Compare/2, "Leak Current, IL"/1, v/1
  I/1 -> Sum/3
  Gain/1 -> Iinter/1, Sum/2

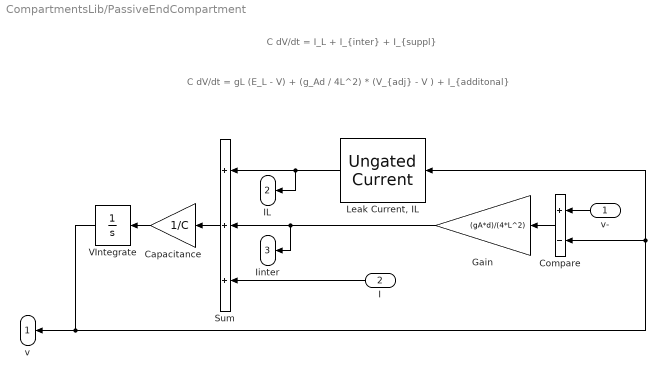
== system CompartmentsLib/PassiveEndCompartment ==
  note: C dV/dt = I_L + I_{inter} + I_{suppl}
  note: C dV/dt = gL (E_L - V) + (g_Ad / 4L^2) * (V_{adj} - V ) + I_{additonal}
  v- : Inport
  I : Inport  Port=2
  Capacitance : Gain  Gain=1/C
  Compare : Sum  Inputs=+-
  Gain : Gain  Gain=(gA*d)/(4*L^2)
  "Leak Current, IL" : CurrentsLib/Ungated Current  SystemSampleTime=-1  EX=EL  gX=gL
  Sum : Sum  Inputs=+++
  VIntegrate : Integrator  InitialCondition=V0
  v : Outport
  IL : Outport  Port=2
  Iinter : Outport  Port=3
  wires:
  Gain/1 -> Sum/2, Iinter/1
  I/1 -> Sum/3
  VIntegrate/1 -> v/1, "Leak Current, IL"/1, Compare/2
  Capacitance/1 -> VIntegrate/1
  Sum/1 -> Capacitance/1
  "Leak Current, IL"/1 -> Sum/1, IL/1
  Compare/1 -> Gain/1
  v-/1 -> Compare/1
